simulink model "hardware_project"  (R2018a)
settings: Solver=FixedStepAuto  StartTime=0.0  StopTime=10  FixedStep=0.00001  RelTol=1e-3
libraries: powerlib x17
settings Model: Creator=nailt  LastModifiedBy=nailt

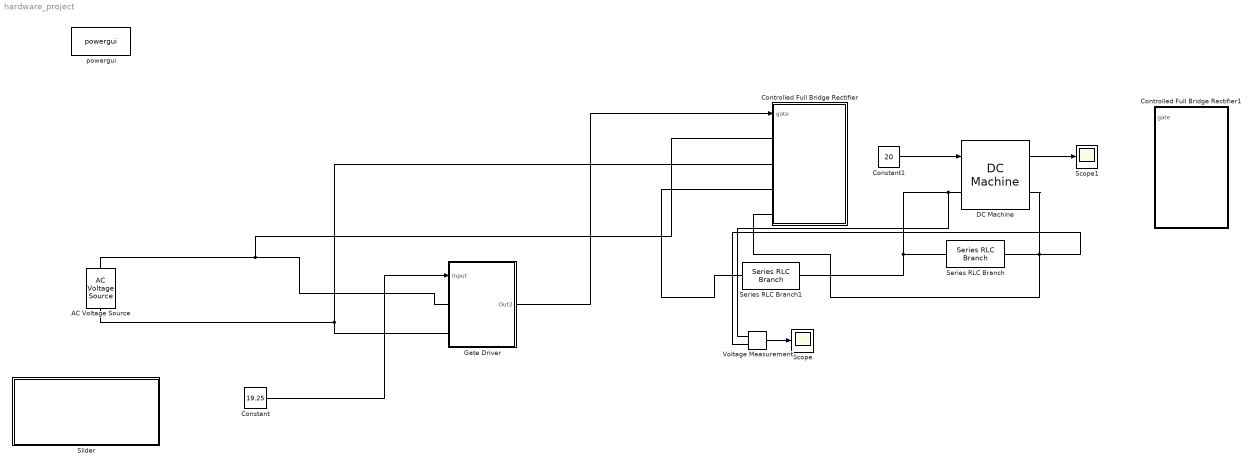
== system hardware_project ==
  AC Voltage Source : powerlib/Electrical Sources/AC Voltage Source  Amplitude=230*sqrt(2)  Phase=0  Frequency=50  SampleTime=0  Measurements=None  BusType=swing  Pref=10e3  Qref=0  Qmin=-inf  Qmax=+inf
  Constant : Constant  Value=19.25
  Constant1 : Constant  Value=20
  Controlled Full Bridge Rectifier : Subsystem
  Controlled Full Bridge Rectifier1 : Subsystem
  DC Machine : powerlib/Machines/DC Machine  PresetModel=No  MechanicalLoad=Torque TL  FieldType=Permanent magnet  ShowDetailedParameters=on  MeasurementBus=on  RLa="[28  0.0133]"  RLf="[ 240  120]"  Laf=1.8  MachineConstant=Back-emf constant (V/rpm)  Ke=1  Kt=1.8  J=1  Bm=0  Tf=0  w0=1  Ifinit=1  TsPowergui=0  TsBlock=-1
  Gate Driver : Subsystem
  Scope : Scope
  Scope1 : Scope
  Series RLC Branch : powerlib/Elements/Series RLC Branch  LConnTagsString=__new0  RConnTagsString=__new0  BranchType=C  Resistance=1  Inductance=1e-3  SetiL0=off  InitialCurrent=0  Capacitance=1e-3  Setx0=off  InitialVoltage=0  Measurements=None
  Series RLC Branch1 : powerlib/Elements/Series RLC Branch  LConnTagsString=__new0  RConnTagsString=__new0  BranchType=L  Resistance=1  Inductance=0.2  SetiL0=off  InitialCurrent=0  Capacitance=1e-6  Setx0=off  InitialVoltage=0  Measurements=None
  Slider : Subsystem  DialogController=hmiCreateDDGDialog  IsWebBlock=on  mask(MWDashboardBlock){webBlockId=14d709ca-2a21-4397-a862-bc9b932952e4, webBlockType=slider, ShowInLibBrowser=on, ShowInitialText=on, HMISrcModelName=hardware_project}
      mask prompts: webBlockId "WebBlock Id"; webBlockType "WebBlock Type"; HMISrcModelName "Source Model"
      mask help: SimulinkHMI:dialogs:SliderDialogDesc
      mask Help: helpview([docroot '/mapfiles/simulink.map'], 'hmi_slider')
      mask Display:
      | if strcmp(get_param(bdroot(gcb),'BlockDiagramType'), 'library')
      |     image([(matlabroot) '/toolbox/simulink/hmi/icons/Slider.png']);
      | end
  Voltage Measurement : powerlib/Measurements/Voltage Measurement  PhasorSimulation=off  OutputType=Complex  PSBequivalent=0
  powergui : powerlib/powergui  Priority=1  SimulationMode=Discrete  SampleTime=0.00001  frequency=60  Iterations=50  frequencyindice=0  Pbase=100e6  ErrMax=1e-4  UnitsV=kV  UnitsW=MW  buscounter=0  FunctionMessages=off  echomessages=off  EnableUseOfTLC=off  CurrentSourceSwitches=off  DisableSnubberDevices=off  DisableRonSwitches=off  DisableVfSwitches=off  DisplayEquations=off  SolverType=Tustin/Backward Euler (TBE)  Interpol=off  ExternalGateDelay=off  methode=off  Ts=100  x0status=blocks  SPID=off  SwTol=0  HookPort=off  RestoreLinks=warning  ResistiveCurrentMeasurement=off  Frange=[0:2:500]  Ylog=off  Xlog=on  ShowGrid=off  save=off  variable=ZData  structure=0  ZoomFFT=off  StartTime=0.0  cycles=1  DisplayStyle=1  fundamental=60  FreqAxis=off  MaxFrequency=1000  frequencyindicesteady=1  RmsSteady=1  display=off
  wires:
  Voltage Measurement/1 -> Scope/1
  Constant/1 -> Gate Driver/1(Input)
  Gate Driver/1(Out2) -> Controlled Full Bridge Rectifier/1(gate)
  Constant1/1 -> DC Machine/1
  DC Machine/1 -> Scope1/1
  connections:
  Gate Driver/LConn1 -- Controlled Full Bridge Rectifier/LConn1 -- AC Voltage Source/RConn1
  Gate Driver/LConn2 -- Controlled Full Bridge Rectifier/LConn2 -- AC Voltage Source/LConn1
  Series RLC Branch1/RConn1 -- Controlled Full Bridge Rectifier/LConn3
  DC Machine/RConn1 -- Voltage Measurement/LConn2 -- Series RLC Branch/RConn1 -- Controlled Full Bridge Rectifier/LConn4
  Series RLC Branch/LConn1 -- Voltage Measurement/LConn1 -- DC Machine/LConn1 -- Series RLC Branch1/LConn1

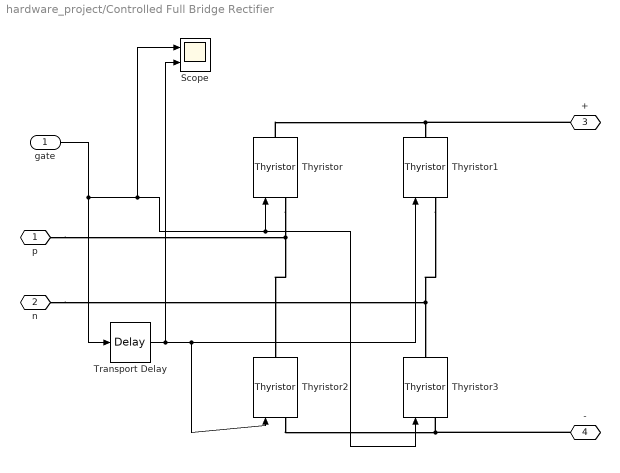
== system hardware_project/Controlled Full Bridge Rectifier ==
  gate : Inport
  Scope : Scope  NumInputPorts=2
  Thyristor{,1..3} (4 alike) : powerlib/Power Electronics/Thyristor  Ron=0.00001  Lon=0  Vf=0  IC=0  Rs=10e9  Cs=250e-12  Measurements=off
  Transport Delay : TransportDelay  DelayTime=0.01
  p : PMIOPort  Side=Left
  n : PMIOPort  Port=2  Side=Left
  + : PMIOPort  Port=3  Side=Left
  - : PMIOPort  Port=4  Side=Left
  wires:
  Transport Delay/1 -> Thyristor1/1, Thyristor2/1, Scope/2
  gate/1 -> Scope/1, Thyristor3/1, Thyristor/1, Transport Delay/1
  connections:
  Thyristor/RConn1 -- +/RConn1 -- Thyristor1/RConn1
  Thyristor/LConn1 -- p/RConn1 -- Thyristor2/RConn1
  Thyristor2/LConn1 -- -/RConn1 -- Thyristor3/LConn1
  Thyristor1/LConn1 -- n/RConn1 -- Thyristor3/RConn1

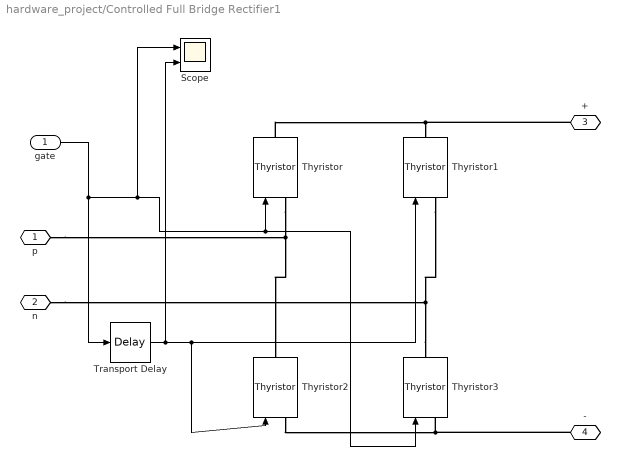
== system hardware_project/Controlled Full Bridge Rectifier1 ==
  gate : Inport
  Scope : Scope  NumInputPorts=2
  Thyristor{,1..3} (4 alike) : powerlib/Power Electronics/Thyristor  Ron=0.00001  Lon=0  Vf=0  IC=0  Rs=10e9  Cs=250e-12  Measurements=off
  Transport Delay : TransportDelay  DelayTime=0.01
  p : PMIOPort  Side=Left
  n : PMIOPort  Port=2  Side=Left
  + : PMIOPort  Port=3  Side=Left
  - : PMIOPort  Port=4  Side=Left
  wires:
  Transport Delay/1 -> Thyristor1/1, Thyristor2/1, Scope/2
  gate/1 -> Scope/1, Thyristor3/1, Thyristor/1, Transport Delay/1
  connections:
  Thyristor/RConn1 -- Thyristor1/RConn1 -- +/RConn1
  Thyristor2/RConn1 -- Thyristor/LConn1 -- p/RConn1
  Thyristor3/LConn1 -- Thyristor2/LConn1 -- -/RConn1
  Thyristor3/RConn1 -- Thyristor1/LConn1 -- n/RConn1

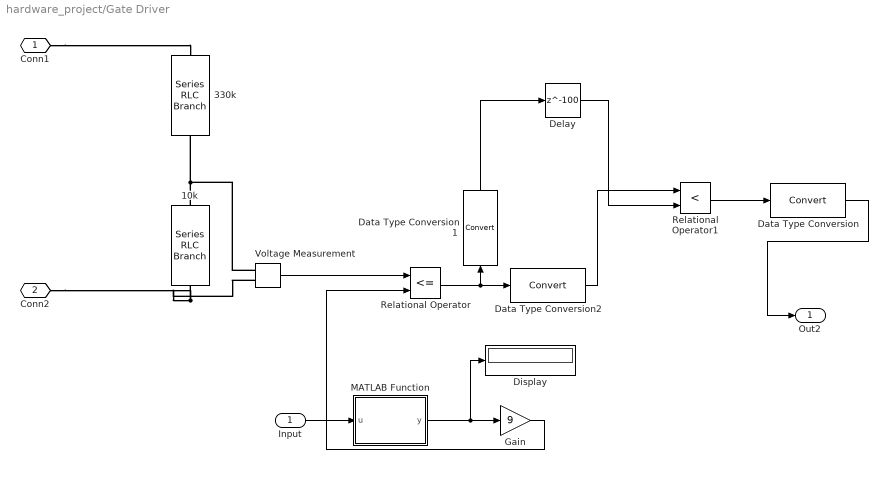
== system hardware_project/Gate Driver ==
  Input : Inport
  10k : powerlib/Elements/Series RLC Branch  LConnTagsString=__new0  RConnTagsString=__new0  BranchType=R  Resistance=10000  Inductance=1e-3  SetiL0=off  InitialCurrent=0  Capacitance=1e-6  Setx0=off  InitialVoltage=0  Measurements=None
  330k : powerlib/Elements/Series RLC Branch  LConnTagsString=__new0  RConnTagsString=__new0  BranchType=R  Resistance=330000  Inductance=1e-3  SetiL0=off  InitialCurrent=0  Capacitance=1e-6  Setx0=off  InitialVoltage=0  Measurements=None
  Data Type Conversion : DataTypeConversion
  Data Type Conversion1 : DataTypeConversion
  Data Type Conversion2 : DataTypeConversion
  Delay : Delay  DelayLength=100
  Display : Display
  Gain : Gain  Gain=9
  MATLAB Function : MATLAB Function  TreatAsAtomicUnit=on
  Relational Operator : RelationalOperator  Operator=<=  OutDataTypeStr=boolean  RndMeth=Simplest
  Relational Operator1 : RelationalOperator  Operator=<  OutDataTypeStr=boolean  RndMeth=Simplest
  Voltage Measurement : powerlib/Measurements/Voltage Measurement  PhasorSimulation=off  OutputType=Complex  PSBequivalent=0
  Conn1 : PMIOPort  Side=Left
  Conn2 : PMIOPort  Port=2  Side=Left
  Out2 : Outport
  wires:
  Voltage Measurement/1 -> Relational Operator/1
  Input/1 -> MATLAB Function/1(u)
  Relational Operator/1 -> Data Type Conversion1/1, Data Type Conversion2/1
  MATLAB Function/1(y) -> Display/1, Gain/1
  Gain/1 -> Relational Operator/2
  Data Type Conversion/1 -> Out2/1
  Relational Operator1/1 -> Data Type Conversion/1
  Data Type Conversion1/1 -> Delay/1
  Delay/1 -> Relational Operator1/2
  Data Type Conversion2/1 -> Relational Operator1/1
  connections:
  10k/RConn1 -- Conn2/RConn1 -- Voltage Measurement/LConn2
  10k/LConn1 -- Voltage Measurement/LConn1 -- 330k/RConn1
  Conn1/RConn1 -- 330k/LConn1

== system hardware_project/Slider ==

== matlab function hardware_project/Gate Driver/MATLAB Function ==
  data: u input; y output
function y = fcn(u)

y = sind(u);
